simulink model "PIDcon"  (Simulink 6.0)
settings: Solver=ode23  StartTime=0.0  StopTime=100.0  RelTol=1e-3
libraries: simulink_extras x1
settings Model: LastModifiedBy=dell
settings OptimizationCC: InlineInvariantSignals=off

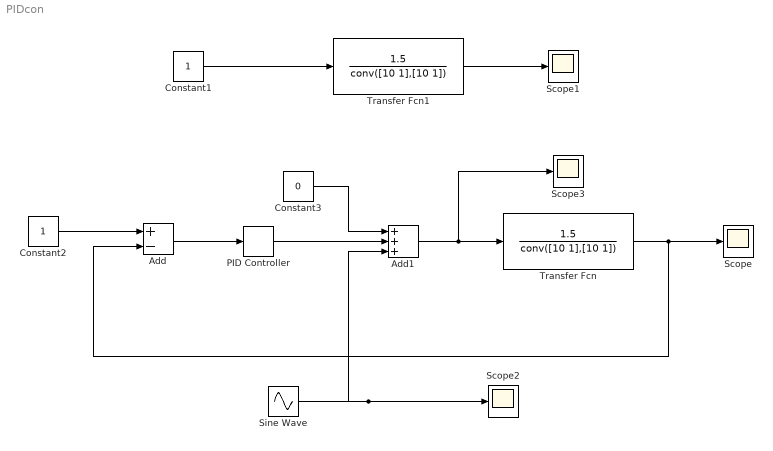
== system PIDcon ==
  Add : Sum  Inputs=+-  OutScaling=2^-10
  Add1 : Sum  Inputs=+++  OutScaling=2^-10
  Constant1 : Constant
  Constant2 : Constant
  Constant3 : Constant  Value=0
  PID Controller : simulink_extras/Additional Linear/PID Controller  P=2  I=0.1  D=0
  Scope{,1..3} (4 alike) : Scope
      Scope2 settings: SaveName=ScopeData2
      Scope3 settings: TimeRange=100  SaveName=ScopeData3
  Sine Wave : Sin  Amplitude=0  SampleTime=0
  Transfer Fcn : TransferFcn  Numerator=[1.5]  Denominator=conv([10 1],[10 1])
  Transfer Fcn1 : TransferFcn  Numerator=[1.5]  Denominator=conv([10 1],[10 1])
  wires:
  Add/1 -> PID Controller/1
  Transfer Fcn/1 -> Scope/1, Add/2
  Constant1/1 -> Transfer Fcn1/1
  Transfer Fcn1/1 -> Scope1/1
  Add1/1 -> Transfer Fcn/1, Scope3/1
  PID Controller/1 -> Add1/2
  Constant3/1 -> Add1/1
  Sine Wave/1 -> Add1/3, Scope2/1
  Constant2/1 -> Add/1
